simulink model "main"  (R2018a)
settings: Solver=VariableStepAuto  StartTime=0.0  StopTime=10.0  RelTol=1e-3
undefined symbols (not defined in the file): DiscIntNeverNeededParam
libraries: simulink x3
settings Model: Creator=henry  LastModifiedBy=henry

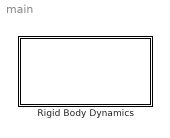
== system main ==
  Rigid Body Dynamics : Subsystem

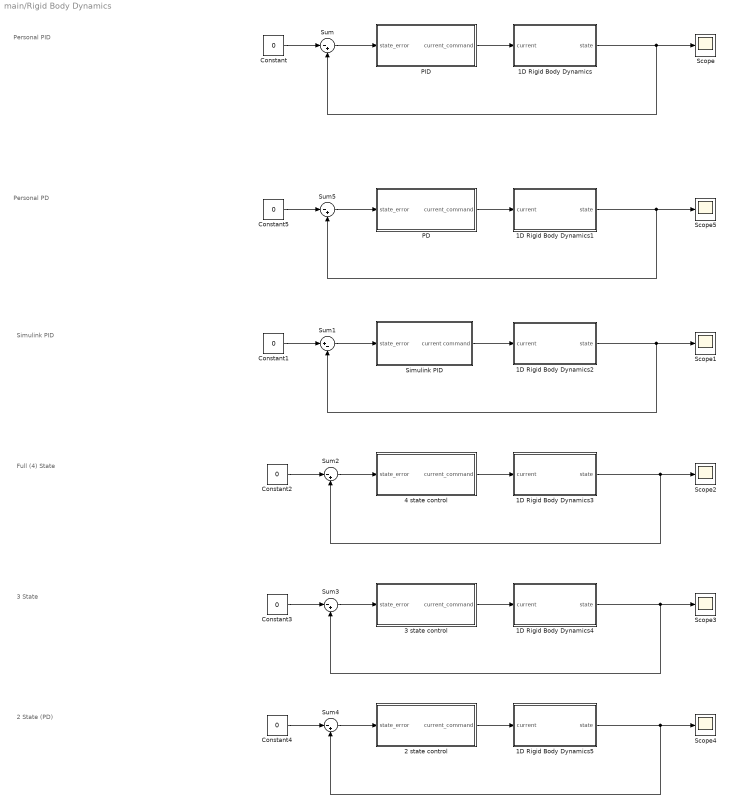
== system main/Rigid Body Dynamics ==
  note: Personal PID
  note: Personal PD
  note: Simulink PID
  note: Full (4) State
  note: 3 State
  note: 2 State (PD)
  1D Rigid Body Dynamics : Subsystem
  1D Rigid Body Dynamics1 : Subsystem
  1D Rigid Body Dynamics2 : Subsystem
  1D Rigid Body Dynamics3 : Subsystem
  1D Rigid Body Dynamics4 : Subsystem
  1D Rigid Body Dynamics5 : Subsystem
  2 state control : Subsystem
  3 state control : Subsystem
  4 state control : Subsystem
  Constant{,1..5} (6 alike) : Constant  Value=0
  PD : Subsystem
  PID : Subsystem
  Scope{,1..5} (6 alike) : Scope
  Simulink PID : Subsystem
  Sum{,2..5} (5 alike) : Sum  Inputs=|-+
  Sum1 : Sum  Inputs=|+-
  wires:
  Constant/1 -> Sum/1
  1D Rigid Body Dynamics/1(state) -> Scope/1, Sum/2
  PID/1(current_command) -> 1D Rigid Body Dynamics/1(current)
  Sum/1 -> PID/1(state_error)
  1D Rigid Body Dynamics2/1(state) -> Scope1/1, Sum1/2
  Constant1/1 -> Sum1/1
  Constant2/1 -> Sum2/1
  1D Rigid Body Dynamics3/1(state) -> Sum2/2, Scope2/1
  Sum2/1 -> 4 state control/1(state_error)
  Sum3/1 -> 3 state control/1(state_error)
  1D Rigid Body Dynamics4/1(state) -> Scope3/1, Sum3/2
  Constant3/1 -> Sum3/1
  Constant4/1 -> Sum4/1
  1D Rigid Body Dynamics5/1(state) -> Scope4/1, Sum4/2
  Sum4/1 -> 2 state control/1(state_error)
  Sum5/1 -> PD/1(state_error)
  PD/1(current_command) -> 1D Rigid Body Dynamics1/1(current)
  1D Rigid Body Dynamics1/1(state) -> Sum5/2, Scope5/1
  Constant5/1 -> Sum5/1
  Simulink PID/1(current command) -> 1D Rigid Body Dynamics2/1(current)
  Sum1/1 -> Simulink PID/1(state_error)
  4 state control/1(current_command) -> 1D Rigid Body Dynamics3/1(current)
  3 state control/1(current_command) -> 1D Rigid Body Dynamics4/1(current)
  2 state control/1(current_command) -> 1D Rigid Body Dynamics5/1(current)

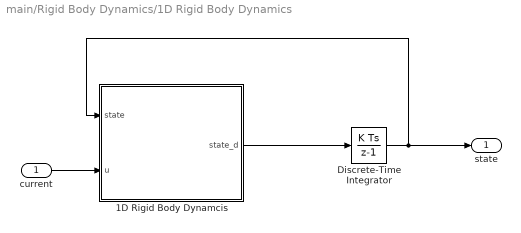
== system main/Rigid Body Dynamics/1D Rigid Body Dynamics ==
  current : Inport
  1D Rigid Body Dynamcis : MATLAB Function  TreatAsAtomicUnit=on
  Discrete-Time Integrator : DiscreteIntegrator  InitialCondition=[0 0 0 0]  SampleTime=-1  ICPrevOutput=DiscIntNeverNeededParam  ICPrevScaledInput=DiscIntNeverNeededParam
  state : Outport
  wires:
  Discrete-Time Integrator/1 -> state/1, 1D Rigid Body Dynamcis/1(state)
  1D Rigid Body Dynamcis/1(state_d) -> Discrete-Time Integrator/1
  current/1 -> 1D Rigid Body Dynamcis/2(u)

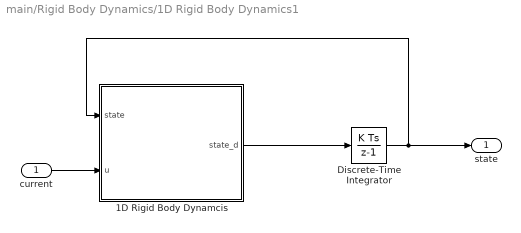
== system main/Rigid Body Dynamics/1D Rigid Body Dynamics1 ==
  current : Inport
  1D Rigid Body Dynamcis : MATLAB Function  TreatAsAtomicUnit=on
  Discrete-Time Integrator : DiscreteIntegrator  InitialCondition=[0 0 0 0]  SampleTime=-1  ICPrevOutput=DiscIntNeverNeededParam  ICPrevScaledInput=DiscIntNeverNeededParam
  state : Outport
  wires:
  current/1 -> 1D Rigid Body Dynamcis/2(u)
  1D Rigid Body Dynamcis/1(state_d) -> Discrete-Time Integrator/1
  Discrete-Time Integrator/1 -> 1D Rigid Body Dynamcis/1(state), state/1

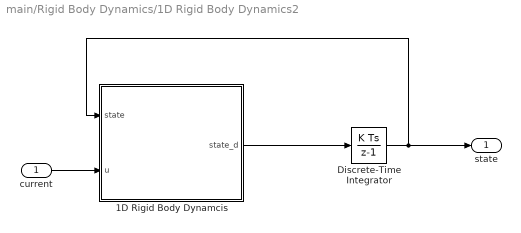
== system main/Rigid Body Dynamics/1D Rigid Body Dynamics2 ==
  current : Inport
  1D Rigid Body Dynamcis : MATLAB Function  TreatAsAtomicUnit=on
  Discrete-Time Integrator : DiscreteIntegrator  InitialCondition=[0 0 0 0]  SampleTime=-1  ICPrevOutput=DiscIntNeverNeededParam  ICPrevScaledInput=DiscIntNeverNeededParam
  state : Outport
  wires:
  Discrete-Time Integrator/1 -> state/1, 1D Rigid Body Dynamcis/1(state)
  1D Rigid Body Dynamcis/1(state_d) -> Discrete-Time Integrator/1
  current/1 -> 1D Rigid Body Dynamcis/2(u)

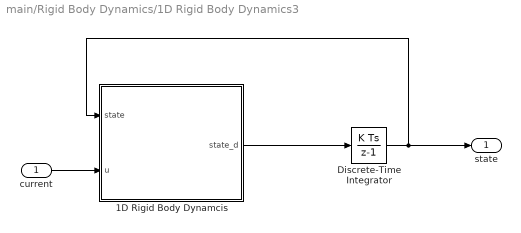
== system main/Rigid Body Dynamics/1D Rigid Body Dynamics3 ==
  current : Inport
  1D Rigid Body Dynamcis : MATLAB Function  TreatAsAtomicUnit=on
  Discrete-Time Integrator : DiscreteIntegrator  InitialCondition=[0 0 0 0]  SampleTime=-1  ICPrevOutput=DiscIntNeverNeededParam  ICPrevScaledInput=DiscIntNeverNeededParam
  state : Outport
  wires:
  current/1 -> 1D Rigid Body Dynamcis/2(u)
  1D Rigid Body Dynamcis/1(state_d) -> Discrete-Time Integrator/1
  Discrete-Time Integrator/1 -> 1D Rigid Body Dynamcis/1(state), state/1

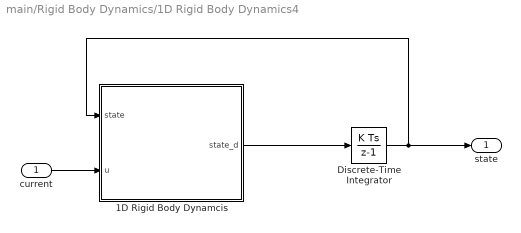
== system main/Rigid Body Dynamics/1D Rigid Body Dynamics4 ==
  current : Inport
  1D Rigid Body Dynamcis : MATLAB Function  TreatAsAtomicUnit=on
  Discrete-Time Integrator : DiscreteIntegrator  InitialCondition=[0 0 0 0]  SampleTime=-1  ICPrevOutput=DiscIntNeverNeededParam  ICPrevScaledInput=DiscIntNeverNeededParam
  state : Outport
  wires:
  Discrete-Time Integrator/1 -> state/1, 1D Rigid Body Dynamcis/1(state)
  1D Rigid Body Dynamcis/1(state_d) -> Discrete-Time Integrator/1
  current/1 -> 1D Rigid Body Dynamcis/2(u)

== system main/Rigid Body Dynamics/1D Rigid Body Dynamics5 ==
  current : Inport
  1D Rigid Body Dynamcis : MATLAB Function  TreatAsAtomicUnit=on
  Discrete-Time Integrator : DiscreteIntegrator  InitialCondition=[0 0 0 0]  SampleTime=-1  ICPrevOutput=DiscIntNeverNeededParam  ICPrevScaledInput=DiscIntNeverNeededParam
  state : Outport
  wires:
  current/1 -> 1D Rigid Body Dynamcis/2(u)
  1D Rigid Body Dynamcis/1(state_d) -> Discrete-Time Integrator/1
  Discrete-Time Integrator/1 -> 1D Rigid Body Dynamcis/1(state), state/1

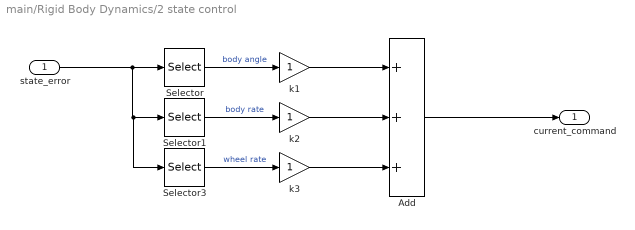
== system main/Rigid Body Dynamics/2 state control ==
  state_error : Inport
  Add : Sum  Inputs=+++
  Selector : Selector  InputPortWidth=4  IndexOptions=Index vector (dialog)  Indices=[1]  OutputSizes=1
  Selector1 : Selector  InputPortWidth=4  IndexOptions=Index vector (dialog)  Indices=[2]  OutputSizes=1
  Selector3 : Selector  InputPortWidth=4  IndexOptions=Index vector (dialog)  Indices=[4]  OutputSizes=1
  k1 : Gain
  k2 : Gain
  k3 : Gain
  current_command : Outport
  wires:
  Add/1 -> current_command/1
  k3/1 -> Add/3
  state_error/1 -> Selector3/1, Selector1/1, Selector/1
  Selector3/1 -> k3/1  "wheel rate"
  Selector1/1 -> k2/1  "body rate"
  Selector/1 -> k1/1  "body angle"
  k1/1 -> Add/1
  k2/1 -> Add/2

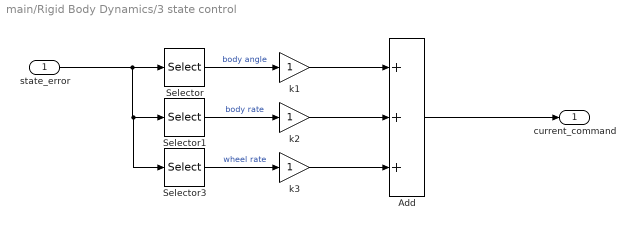
== system main/Rigid Body Dynamics/3 state control ==
  state_error : Inport
  Add : Sum  Inputs=+++
  Selector : Selector  InputPortWidth=4  IndexOptions=Index vector (dialog)  Indices=[1]  OutputSizes=1
  Selector1 : Selector  InputPortWidth=4  IndexOptions=Index vector (dialog)  Indices=[2]  OutputSizes=1
  Selector3 : Selector  InputPortWidth=4  IndexOptions=Index vector (dialog)  Indices=[4]  OutputSizes=1
  k1 : Gain
  k2 : Gain
  k3 : Gain
  current_command : Outport
  wires:
  k2/1 -> Add/2
  k1/1 -> Add/1
  Selector/1 -> k1/1  "body angle"
  Selector1/1 -> k2/1  "body rate"
  Selector3/1 -> k3/1  "wheel rate"
  state_error/1 -> Selector/1, Selector1/1, Selector3/1
  k3/1 -> Add/3
  Add/1 -> current_command/1

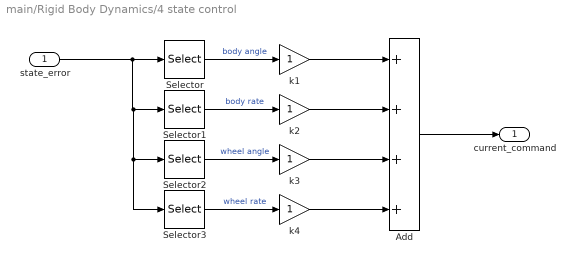
== system main/Rigid Body Dynamics/4 state control ==
  state_error : Inport
  Add : Sum  Inputs=++++
  Selector : Selector  InputPortWidth=4  IndexOptions=Index vector (dialog)  Indices=[1]  OutputSizes=1
  Selector1 : Selector  InputPortWidth=4  IndexOptions=Index vector (dialog)  Indices=[2]  OutputSizes=1
  Selector2 : Selector  InputPortWidth=4  IndexOptions=Index vector (dialog)  Indices=[3]  OutputSizes=1
  Selector3 : Selector  InputPortWidth=4  IndexOptions=Index vector (dialog)  Indices=[4]  OutputSizes=1
  k{1..4} (4 alike) : Gain
  current_command : Outport
  wires:
  state_error/1 -> Selector3/1, Selector2/1, Selector1/1, Selector/1
  Selector3/1 -> k4/1  "wheel rate"
  Selector2/1 -> k3/1  "wheel angle"
  Selector1/1 -> k2/1  "body rate"
  Selector/1 -> k1/1  "body angle"
  k1/1 -> Add/1
  k2/1 -> Add/2
  k4/1 -> Add/4
  k3/1 -> Add/3
  Add/1 -> current_command/1

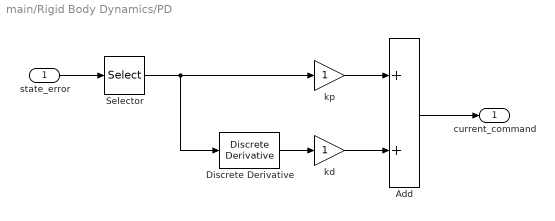
== system main/Rigid Body Dynamics/PD ==
  state_error : Inport
  Add : Sum
  Discrete Derivative : simulink/Discrete/Discrete Derivative  gainval=1.0  ICPrevScaledInput=0.0  OutMin=[]  OutMax=[]  OutDataType=fixdt(1, 16)  OutScaling=2^-10  DoSatur=off
  Selector : Selector  InputPortWidth=4  IndexOptions=Index vector (dialog)  Indices=[1]  OutputSizes=1
  kd : Gain
  kp : Gain
  current_command : Outport
  wires:
  Add/1 -> current_command/1
  Selector/1 -> kp/1, Discrete Derivative/1
  Discrete Derivative/1 -> kd/1
  state_error/1 -> Selector/1
  kp/1 -> Add/1
  kd/1 -> Add/2

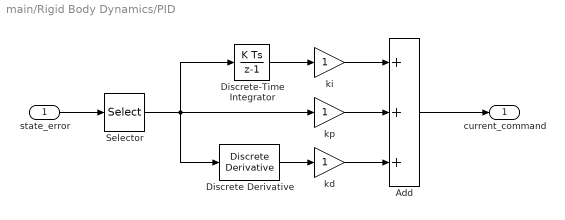
== system main/Rigid Body Dynamics/PID ==
  state_error : Inport
  Add : Sum  Inputs=+++
  Discrete Derivative : simulink/Discrete/Discrete Derivative  gainval=1.0  ICPrevScaledInput=0.0  OutMin=[]  OutMax=[]  OutDataType=fixdt(1, 16)  OutScaling=2^-10  DoSatur=off
  Discrete-Time Integrator : DiscreteIntegrator  SampleTime=-1  ICPrevOutput=DiscIntNeverNeededParam  ICPrevScaledInput=DiscIntNeverNeededParam
  Selector : Selector  InputPortWidth=4  IndexOptions=Index vector (dialog)  Indices=[1]  OutputSizes=1
  kd : Gain
  ki : Gain
  kp : Gain
  current_command : Outport
  wires:
  state_error/1 -> Selector/1
  Discrete-Time Integrator/1 -> ki/1
  Discrete Derivative/1 -> kd/1
  Selector/1 -> Discrete Derivative/1, kp/1, Discrete-Time Integrator/1
  kp/1 -> Add/2
  Add/1 -> current_command/1
  kd/1 -> Add/3
  ki/1 -> Add/1

== system main/Rigid Body Dynamics/Simulink PID ==
  state_error : Inport
  Discrete PID Controller : simulink/Continuous/PID Controller  Controller=PID  TimeDomain=Discrete-time  SampleTime=-1  IntegratorMethod=Forward Euler  FilterMethod=Forward Euler  Form=Parallel  UseFilter=on  ControllerParametersSource=internal  P=1  I=1  D=0  N=100  InitialConditionSource=internal  InitialConditionForIntegrator=0  InitialConditionForFilter=0  ExternalReset=none  LimitOutput=off  UpperSaturationLimit=inf  LowerSaturationLimit=-inf  LinearizeAsGain=off  AntiWindupMode=none  Kb=1  TrackingMode=off  Kt=1  PParamMin=[]  PParamMax=[]  IParamMin=[]  IParamMax=[]  DParamMin=[]  DParamMax=[]  NParamMin=[]  NParamMax=[]  KbParamMin=[]  KbParamMax=[]  KtParamMin=[]  KtParamMax=[]  POutMin=[]  POutMax=[]  IOutMin=[]  IOutMax=[]  DOutMin=[]  DOutMax=[]  NOutMin=[]  NOutMax=[]  KbOutMin=[]  KbOutMax=[]  KtOutMin=[]  KtOutMax=[]  IntegratorOutMin=[]  IntegratorOutMax=[]  FilterOutMin=[]  FilterOutMax=[]  SumOutMin=[]  SumOutMax=[]  SumI1OutMin=[]  SumI1OutMax=[]  SumI2OutMin=[]  SumI2OutMax=[]  SumI3OutMin=[]  SumI3OutMax=[]  SumDOutMin=[]  SumDOutMax=[]  SaturationOutMin=[]  SaturationOutMax=[]  IntegratorContinuousStateAttributes=''  IntegratorStateMustResolveToSignalObject=off  IntegratorRTWStateStorageClass=Auto  FilterContinuousStateAttributes=''  FilterStateMustResolveToSignalObject=off  FilterRTWStateStorageClass=Auto  DifferentiatorICPrevScaledInput=0  DifferentiatorOutMin=[]  DifferentiatorOutMax=[]  FilterDiffOutCoefMin=[]  FilterDiffOutCoefMax=[]  SumDenOutMin=[]  SumDenOutMax=[]  SumNumOutMin=[]  SumNumOutMax=[]  ReciprocalOutMin=[]  ReciprocalOutMax=[]  DivideOutMin=[]  DivideOutMax=[]  TunerSelectOption=Transfer Function Based (PID Tuner App)
  Selector : Selector  InputPortWidth=4  IndexOptions=Index vector (dialog)  Indices=[1]  OutputSizes=1
  current command : Outport
  wires:
  state_error/1 -> Selector/1
  Selector/1 -> Discrete PID Controller/1
  Discrete PID Controller/1 -> current command/1

== matlab function main/Rigid Body Dynamics/1D Rigid Body Dynamics1/1D Rigid Body Dynamcis ==
  data: state input; u input; state_d output
function state_d = dynamics_1d(state, u)
state_d = zeros(4,1);

l=.085;%m
lb=.075;%m
mb=.419;%kg
mw=.204;%kg
Ib=3.34*10^-3;
Iw=.57*10^-3;
Cb=1.02*10^-3;
Cw=.05*10^-3;
g=9.81;
k=25.1*10^-3;

theta_b=state(1);
theta_bdot=state(2);
theta_wdot=state(4);

f1=theta_bdot;
f2=((mb*lb+mw*l)*g*sin(theta_b)-k*u-Cb*theta_bdot+Cw*theta_wdot)/(Ib+mw*l^2);
f3=theta_wdot;
f4=(Ib+Iw+mw*l^2)*(k*u-Cw*theta_wdot)/(Iw*(Ib+mw*l^2))-((mb*lb+mw*l)*g*sin(theta_b)-Cb*theta_bdot)/(Ib+mw*l^2);

state_d(1) = f1;
state_d(2) = f2;
state_d(3) = f3;
state_d(4) = f4;

end

== matlab function main/Rigid Body Dynamics/1D Rigid Body Dynamics/1D Rigid Body Dynamcis ==
  data: state input; u input; state_d output
function state_d = dynamics_1d(state, u)
state_d = zeros(4,1);

l=.085;%m
lb=.075;%m
mb=.419;%kg
mw=.204;%kg
Ib=3.34*10^-3;
Iw=.57*10^-3;
Cb=1.02*10^-3;
Cw=.05*10^-3;
g=9.81;
k=25.1*10^-3;

theta_b=state(1);
theta_bdot=state(2);
theta_wdot=state(4);

f1=theta_bdot;
f2=((mb*lb+mw*l)*g*sin(theta_b)-k*u-Cb*theta_bdot+Cw*theta_wdot)/(Ib+mw*l^2);
f3=theta_wdot;
f4=(Ib+Iw+mw*l^2)*(k*u-Cw*theta_wdot)/(Iw*(Ib+mw*l^2))-((mb*lb+mw*l)*g*sin(theta_b)-Cb*theta_bdot)/(Ib+mw*l^2);

state_d(1) = f1;
state_d(2) = f2;
state_d(3) = f3;
state_d(4) = f4;

end

== matlab function main/Rigid Body Dynamics/1D Rigid Body Dynamics2/1D Rigid Body Dynamcis ==
  data: state input; u input; state_d output
function state_d = dynamics_1d(state, u)
state_d = zeros(4,1);

l=.085;%m
lb=.075;%m
mb=.419;%kg
mw=.204;%kg
Ib=3.34*10^-3;
Iw=.57*10^-3;
Cb=1.02*10^-3;
Cw=.05*10^-3;
g=9.81;
k=25.1*10^-3;

theta_b=state(1);
theta_bdot=state(2);
theta_wdot=state(4);

f1=theta_bdot;
f2=((mb*lb+mw*l)*g*sin(theta_b)-k*u-Cb*theta_bdot+Cw*theta_wdot)/(Ib+mw*l^2);
f3=theta_wdot;
f4=(Ib+Iw+mw*l^2)*(k*u-Cw*theta_wdot)/(Iw*(Ib+mw*l^2))-((mb*lb+mw*l)*g*sin(theta_b)-Cb*theta_bdot)/(Ib+mw*l^2);

state_d(1) = f1;
state_d(2) = f2;
state_d(3) = f3;
state_d(4) = f4;

end

== matlab function main/Rigid Body Dynamics/1D Rigid Body Dynamics3/1D Rigid Body Dynamcis ==
  data: state input; u input; state_d output
function state_d = dynamics_1d(state, u)
state_d = zeros(4,1);

l=.085;%m
lb=.075;%m
mb=.419;%kg
mw=.204;%kg
Ib=3.34*10^-3;
Iw=.57*10^-3;
Cb=1.02*10^-3;
Cw=.05*10^-3;
g=9.81;
k=25.1*10^-3;

theta_b=state(1);
theta_bdot=state(2);
theta_wdot=state(4);

f1=theta_bdot;
f2=((mb*lb+mw*l)*g*sin(theta_b)-k*u-Cb*theta_bdot+Cw*theta_wdot)/(Ib+mw*l^2);
f3=theta_wdot;
f4=(Ib+Iw+mw*l^2)*(k*u-Cw*theta_wdot)/(Iw*(Ib+mw*l^2))-((mb*lb+mw*l)*g*sin(theta_b)-Cb*theta_bdot)/(Ib+mw*l^2);

state_d(1) = f1;
state_d(2) = f2;
state_d(3) = f3;
state_d(4) = f4;

end

== matlab function main/Rigid Body Dynamics/1D Rigid Body Dynamics4/1D Rigid Body Dynamcis ==
  data: state input; u input; state_d output
function state_d = dynamics_1d(state, u)
state_d = zeros(4,1);

l=.085;%m
lb=.075;%m
mb=.419;%kg
mw=.204;%kg
Ib=3.34*10^-3;
Iw=.57*10^-3;
Cb=1.02*10^-3;
Cw=.05*10^-3;
g=9.81;
k=25.1*10^-3;

theta_b=state(1);
theta_bdot=state(2);
theta_wdot=state(4);

f1=theta_bdot;
f2=((mb*lb+mw*l)*g*sin(theta_b)-k*u-Cb*theta_bdot+Cw*theta_wdot)/(Ib+mw*l^2);
f3=theta_wdot;
f4=(Ib+Iw+mw*l^2)*(k*u-Cw*theta_wdot)/(Iw*(Ib+mw*l^2))-((mb*lb+mw*l)*g*sin(theta_b)-Cb*theta_bdot)/(Ib+mw*l^2);

state_d(1) = f1;
state_d(2) = f2;
state_d(3) = f3;
state_d(4) = f4;

end

== matlab function main/Rigid Body Dynamics/1D Rigid Body Dynamics5/1D Rigid Body Dynamcis ==
  data: state input; u input; state_d output
function state_d = dynamics_1d(state, u)
state_d = zeros(4,1);

l=.085;%m
lb=.075;%m
mb=.419;%kg
mw=.204;%kg
Ib=3.34*10^-3;
Iw=.57*10^-3;
Cb=1.02*10^-3;
Cw=.05*10^-3;
g=9.81;
k=25.1*10^-3;

theta_b=state(1);
theta_bdot=state(2);
theta_wdot=state(4);

f1=theta_bdot;
f2=((mb*lb+mw*l)*g*sin(theta_b)-k*u-Cb*theta_bdot+Cw*theta_wdot)/(Ib+mw*l^2);
f3=theta_wdot;
f4=(Ib+Iw+mw*l^2)*(k*u-Cw*theta_wdot)/(Iw*(Ib+mw*l^2))-((mb*lb+mw*l)*g*sin(theta_b)-Cb*theta_bdot)/(Ib+mw*l^2);

state_d(1) = f1;
state_d(2) = f2;
state_d(3) = f3;
state_d(4) = f4;

end
